simulink model "open_loop_algorithm"  (R2025b)
settings: Solver=FixedStepAuto  StartTime=0.0  StopTime=10.0  RelTol=1e-3  EnableMultiTasking=on
InitFcn:
  | open_loop_data;
values from neighbouring files (symbols this model uses):
  Ts = T_pwm    (= 5e-05)    [open_loop_data.m]
undefined symbols (not defined in the file or in its folder): DiscIntNeverNeededParam, motor
libraries: mcbcontrolslib x2

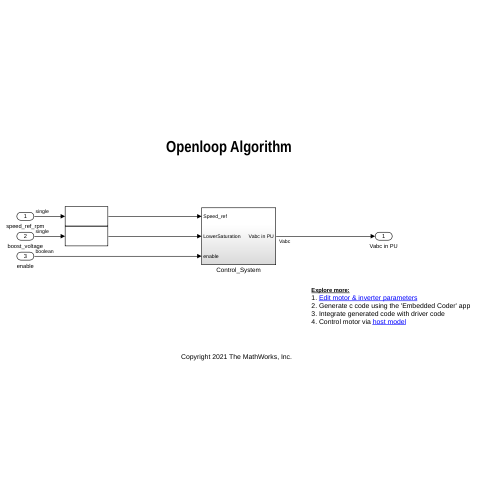
[thumbnail: Simulink's stored preview of the top-level diagram]
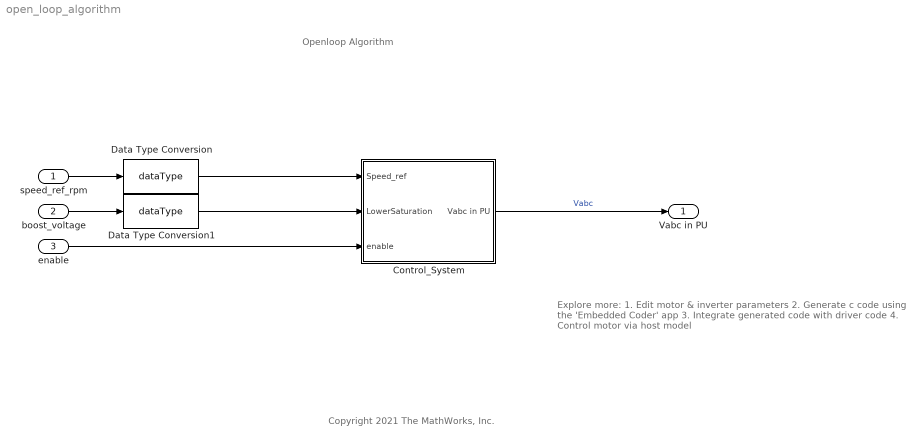
== system open_loop_algorithm ==
  note: Openloop Algorithm
  note: Explore more:
      | 1. Edit motor & inverter parameters
      | 2. Generate c code using the 'Embedded Coder' app
      | 3. Integrate generated code with driver code
      | 4. Control motor via host model
  note: Copyright 2021 The MathWorks, Inc.
  speed_ref_rpm : Inport  OutDataTypeStr=single  PortDimensions=1
  boost_voltage : Inport  Port=2  OutDataTypeStr=single  PortDimensions=1
  enable : Inport  Port=3  OutDataTypeStr=boolean  PortDimensions=1
  Control_System : Subsystem
  Data Type Conversion : DataTypeConversion  OutDataTypeStr=dataType  SaturateOnIntegerOverflow=off  RndMeth=Floor
  Data Type Conversion1 : DataTypeConversion  OutDataTypeStr=dataType  SaturateOnIntegerOverflow=off  RndMeth=Floor
  Vabc in PU : Outport
  wires:
  boost_voltage/1 -> Data Type Conversion1/1
  speed_ref_rpm/1 -> Data Type Conversion/1
  Data Type Conversion/1 -> Control_System/1(Speed_ref)
  Data Type Conversion1/1 -> Control_System/2(LowerSaturation)
  enable/1 -> Control_System/3(enable)
  Control_System/1(Vabc in PU) -> Vabc in PU/1  "Vabc"

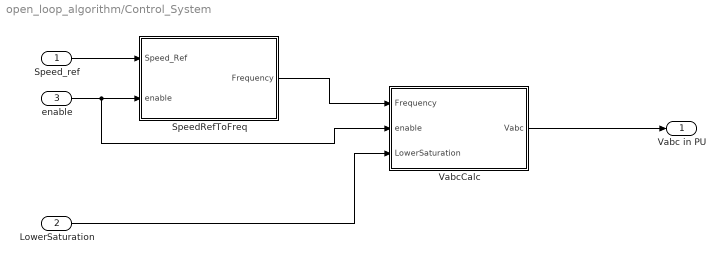
== system open_loop_algorithm/Control_System ==
  Speed_ref : Inport
  LowerSaturation : Inport  Port=2
  enable : Inport  Port=3
  SpeedRefToFreq : Subsystem
  VabcCalc : Subsystem
  Vabc in PU : Outport  VectorParamsAs1DForOutWhenUnconnected=off
  wires:
  Speed_ref/1 -> SpeedRefToFreq/1(Speed_Ref)
  SpeedRefToFreq/1(Frequency) -> VabcCalc/1(Frequency)
  VabcCalc/1(Vabc) -> Vabc in PU/1
  LowerSaturation/1 -> VabcCalc/3(LowerSaturation)
  enable/1 -> VabcCalc/2(enable), SpeedRefToFreq/2(enable)

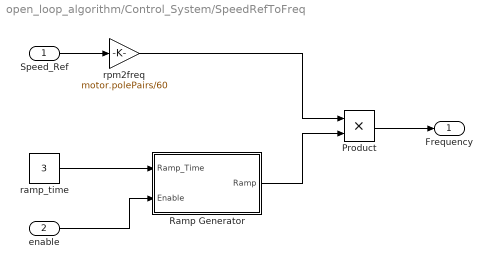
== system open_loop_algorithm/Control_System/SpeedRefToFreq ==
  Speed_Ref : Inport
  enable : Inport  Port=2  OutDataTypeStr=boolean
  Product : Product  RndMeth=Simplest  OutDataTypeStr=Inherit: Same as first input
  Ramp Generator : Subsystem
  ramp_time : Constant  Value=3  OutDataTypeStr=dataType  SampleTime=-1
  rpm2freq : Gain  Gain=motor.polePairs/60  OutDataTypeStr=dataType  RndMeth=Simplest
  Frequency : Outport
  wires:
  Product/1 -> Frequency/1
  Ramp Generator/1(Ramp) -> Product/2
  ramp_time/1 -> Ramp Generator/1(Ramp_Time)
  enable/1 -> Ramp Generator/2(Enable)
  Speed_Ref/1 -> rpm2freq/1
  rpm2freq/1 -> Product/1

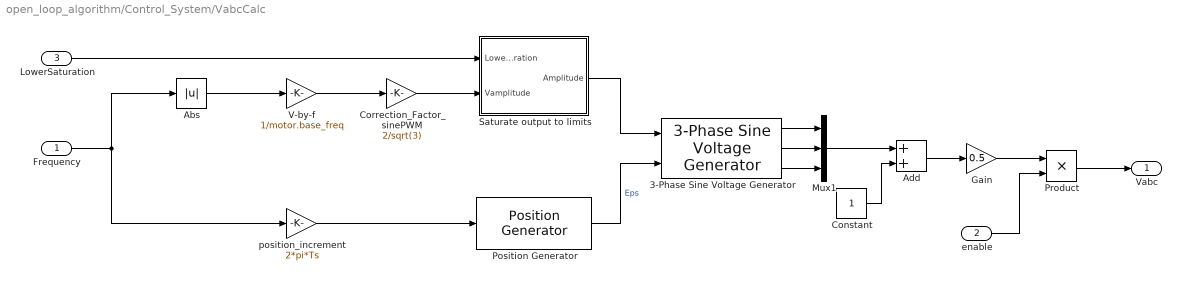
== system open_loop_algorithm/Control_System/VabcCalc ==
  Frequency : Inport
  enable : Inport  Port=2
  LowerSaturation : Inport  Port=3
  3-Phase Sine Voltage Generator : mcbcontrolslib/3-Phase Sine Voltage Generator  AngleInput=Per-unit  N_points=1024
  Abs : Abs  RndMeth=Simplest  SaturateOnIntegerOverflow=off
  Add : Sum
  Constant : Constant  OutDataTypeStr=dataType
  Correction_Factor_sinePWM : Gain  Gain=2/sqrt(3)  RndMeth=Simplest  OutDataTypeStr=Inherit: Same as input
  Gain : Gain  Gain=0.5  RndMeth=Simplest  OutDataTypeStr=Inherit: Same as input
  Mux1 : Mux  Inputs=3
  Position Generator : mcbcontrolslib/Position Generator  AngleOutput=Per-unit  InitialThetaSource=Specify via dialog  ExternalReset=none  Offset=0
  Product : Product  OutDataTypeStr=Inherit: Same as first input
  Saturate output to limits : Subsystem
  V-by-f : Gain  Gain=1/motor.base_freq  RndMeth=Simplest  OutDataTypeStr=Inherit: Same as input
  position_increment : Gain  Gain=2*pi*Ts  RndMeth=Simplest  OutDataTypeStr=Inherit: Same as input
  Vabc : Outport
  wires:
  Frequency/1 -> Abs/1, position_increment/1
  position_increment/1 -> Position Generator/1
  3-Phase Sine Voltage Generator/3 -> Mux1/3
  3-Phase Sine Voltage Generator/2 -> Mux1/2
  V-by-f/1 -> Correction_Factor_sinePWM/1
  3-Phase Sine Voltage Generator/1 -> Mux1/1
  Correction_Factor_sinePWM/1 -> Saturate output to limits/2(Vamplitude)
  LowerSaturation/1 -> Saturate output to limits/1(Lower Saturation)
  Saturate output to limits/1(Amplitude) -> 3-Phase Sine Voltage Generator/1
  Position Generator/1 -> 3-Phase Sine Voltage Generator/2  "Eps"
  Abs/1 -> V-by-f/1
  enable/1 -> Product/2
  Product/1 -> Vabc/1
  Mux1/1 -> Add/1
  Constant/1 -> Add/2
  Add/1 -> Gain/1
  Gain/1 -> Product/1

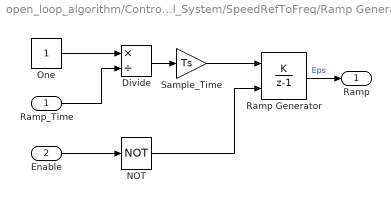
== system open_loop_algorithm/Control_System/SpeedRefToFreq/Ramp Generator ==
  Ramp_Time : Inport
  Enable : Inport  Port=2
  Divide : Product  Inputs=*/  RndMeth=Simplest  OutDataTypeStr=Inherit: Same as first input
  NOT : Logic  Operator=NOT  IconShape=distinctive  AllPortsSameDT=off  OutDataTypeStr=boolean
  One : Constant  OutDataTypeStr=dataType  SampleTime=-1
  Ramp Generator : DiscreteIntegrator  IntegratorMethod=Accumulation: Forward Euler  gainval=1  ExternalReset=sampled level  SampleTime=-1  OutDataTypeStr=dataType  RndMeth=Simplest  LimitOutput=on  UpperSaturationLimit=1  LowerSaturationLimit=0  ICPrevOutput=DiscIntNeverNeededParam  ICPrevScaledInput=DiscIntNeverNeededParam
  Sample_Time : Gain  Gain=Ts  RndMeth=Simplest  OutDataTypeStr=Inherit: Same as input
  Ramp : Outport
  wires:
  Divide/1 -> Sample_Time/1
  Ramp Generator/1 -> Ramp/1  "Eps"
  Sample_Time/1 -> Ramp Generator/1
  One/1 -> Divide/1
  Ramp_Time/1 -> Divide/2
  Enable/1 -> NOT/1
  NOT/1 -> Ramp Generator/2

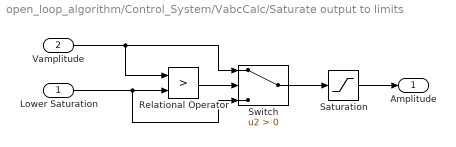
== system open_loop_algorithm/Control_System/VabcCalc/Saturate output to limits ==
  Lower Saturation : Inport
  Vamplitude : Inport  Port=2
  Relational Operator : RelationalOperator  Operator=>  OutDataTypeStr=boolean  RndMeth=Simplest  InputSameDT=off
  Saturation : Saturate  UpperLimit=0.95  LowerLimit=0  RndMeth=Simplest
  Switch : Switch  Criteria=u2 > Threshold  SaturateOnIntegerOverflow=off  InputSameDT=off
  Amplitude : Outport
  wires:
  Saturation/1 -> Amplitude/1
  Switch/1 -> Saturation/1
  Relational Operator/1 -> Switch/2
  Lower Saturation/1 -> Switch/3, Relational Operator/2
  Vamplitude/1 -> Switch/1, Relational Operator/1
